simulink model "senario_1"  (R2023a)
settings: Solver=VariableStepAuto  StartTime=0.0  StopTime=30  RelTol=1e-3
values from neighbouring files (symbols this model uses):
  K = K_ft    (= 60)    [DC_Motor_FLC.m]    (also in DC_Motor_FLC_senario2.m; DC_Motor_FLC_senario3.m)
  Kd = Kd_ft    (= 2)    [DC_Motor_FLC.m]    (also in DC_Motor_FLC_senario2.m; DC_Motor_FLC_senario3.m)
  Ke = Ke_ft    (= 1)    [DC_Motor_FLC.m]    (also in DC_Motor_FLC_senario2.m; DC_Motor_FLC_senario3.m)
  normalization = 1/r_max    (= 0.00666666666667)    [DC_Motor_FLC.m]    (also in DC_Motor_FLC_senario2.m)
  r_max = 150    [DC_Motor_FLC.m]    (also in DC_Motor_FLC_senario2.m)
  Ts = 0.01    [DC_Motor_FLC.m]    (also in DC_Motor_FLC_senario2.m; DC_Motor_FLC_senario3.m)
libraries: fuzblock x1
settings Model: Creator=xkoun  LastModifiedBy=xkoun
settings DataIOCC: ReturnWorkspaceOutputs=off

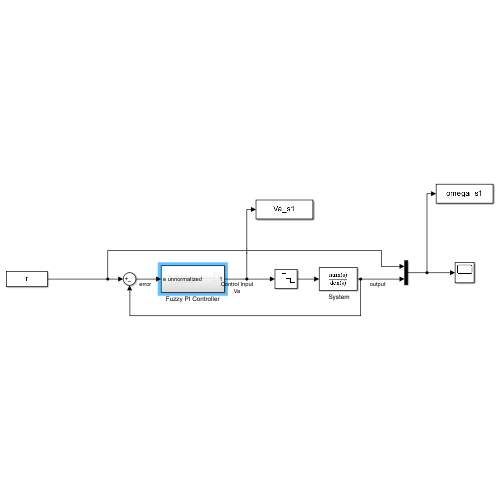
[thumbnail: Simulink's stored preview of the top-level diagram]
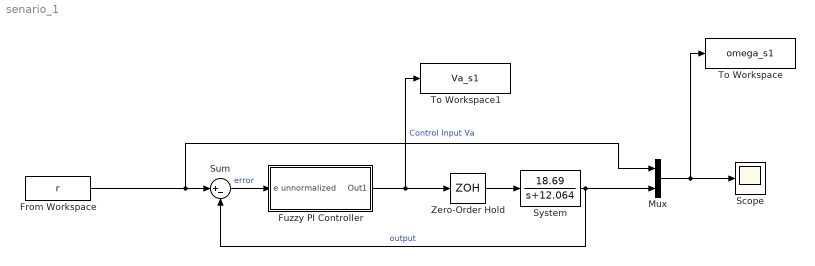
== system senario_1 ==
  " System" : TransferFcn  Numerator=[18.69]  Denominator=[1 12.064]
  From Workspace : FromWorkspace  VariableName=r  SampleTime=Ts
  Fuzzy PI Controller : Subsystem
  Mux : Mux  Inputs=2
  Scope : Scope
  Sum : Sum  Inputs=|+-
  To Workspace : ToWorkspace  VariableName=omega_s1  SaveFormat=Timeseries  SampleTime=-1
  To Workspace1 : ToWorkspace  VariableName=Va_s1  SaveFormat=Timeseries  SampleTime=-1
  Zero-Order Hold : ZeroOrderHold  SampleTime=Ts
  wires:
  From Workspace/1 -> Mux/1, Sum/1
  Sum/1 -> Fuzzy PI Controller/1(e unnormalized)  "error"
  Fuzzy PI Controller/1(Out1) -> To Workspace1/1, Zero-Order Hold/1  "Control Input Va"
  Zero-Order Hold/1 -> " System"/1
  " System"/1 -> Sum/2, Mux/2  "output"
  Mux/1 -> To Workspace/1, Scope/1

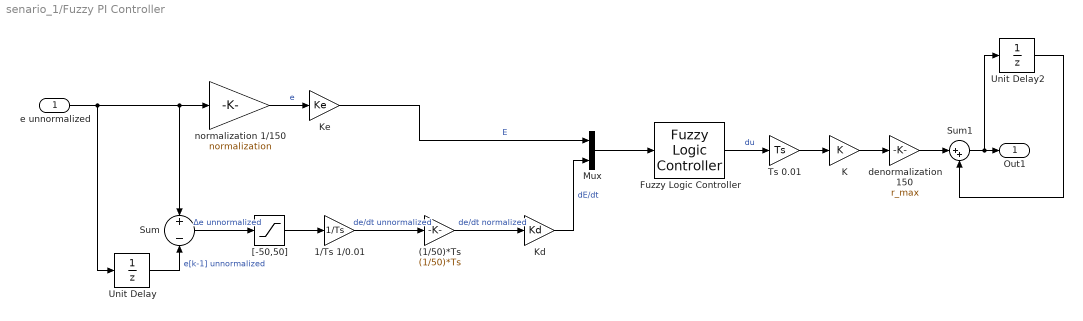
== system senario_1/Fuzzy PI Controller ==
  e unnormalized : Inport
  (1/50)*Ts : Gain  Gain=(1/50)*Ts
  1/Ts 1/0.01 : Gain  Gain=1/Ts
  Fuzzy Logic Controller : fuzblock/Fuzzy Logic  Controller  FIS=fis  OutputSampleNumber=101  DataType=double  FuzzifiedInputs=off  RuleFiringStrengths=off  RuleOutputs=off  AggregatedOutputs=off  SimulateUsing=Interpreted execution  OutOfRangeInputValueMessage=warning  NoRuleFiredMessage=warning  EmptyOutputFuzzySetMessage=warning
  K : Gain  Gain=K
  "Kd " : Gain  Gain=Kd
  "Ke " : Gain  Gain=Ke
  Mux : Mux  Inputs=2
  Sum : Sum  Inputs=+|-
  Sum1 : Sum  Inputs=|++
  Ts 0.01 : Gain  Gain=Ts
  Unit Delay : UnitDelay  SampleTime=Ts  HasFrameUpgradeWarning=on
  Unit Delay2 : UnitDelay  SampleTime=-1  HasFrameUpgradeWarning=on
  "[-50,50]" : Saturate  UpperLimit=50  LowerLimit=-50
  denormalization 150 : Gain  Gain=r_max
  normalization 1/150 : Gain  Gain=normalization
  Out1 : Outport
  wires:
  e unnormalized/1 -> Unit Delay/1, normalization 1/150/1, Sum/1
  Mux/1 -> Fuzzy Logic Controller/1
  Sum1/1 -> Unit Delay2/1, Out1/1
  normalization 1/150/1 -> "Ke "/1  "e"
  Unit Delay/1 -> Sum/2  "e[k-1] unnormalized"
  denormalization 150/1 -> Sum1/1
  Ts 0.01/1 -> K/1
  Fuzzy Logic Controller/1 -> Ts 0.01/1  "du"
  Sum/1 -> "[-50,50]"/1  "Δe unnormalized"
  "Kd "/1 -> Mux/2  "dE/dt"
  "Ke "/1 -> Mux/1  "E"
  K/1 -> denormalization 150/1
  Unit Delay2/1 -> Sum1/2
  (1/50)*Ts/1 -> "Kd "/1  "de/dt normalized"
  "[-50,50]"/1 -> 1/Ts 1/0.01/1
  1/Ts 1/0.01/1 -> (1/50)*Ts/1  "de/dt unnormalized"
